simulink model "untitled"  (R2023a)
settings: Solver=VariableStepAuto  StartTime=0.0  StopTime=25  RelTol=1e-3
libraries: simulink x2
settings Model: Creator=4epe3  LastModifiedBy=4epe3

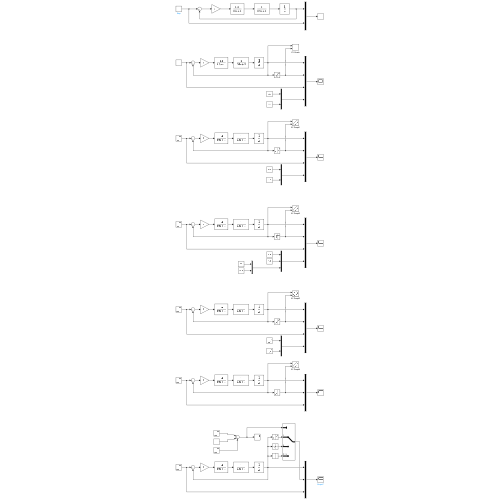
[thumbnail: Simulink's stored preview of the top-level diagram]
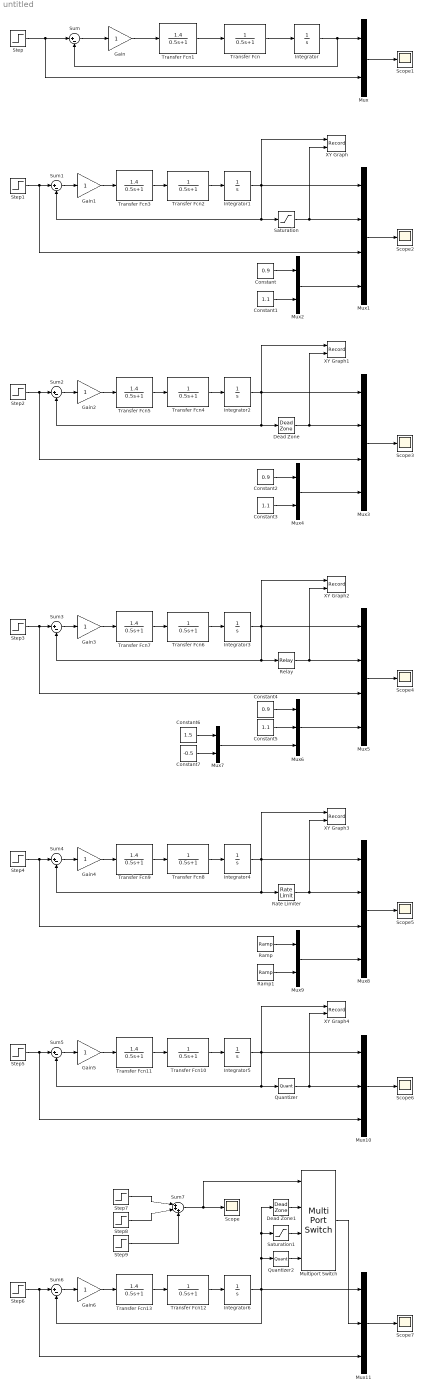
== system untitled ==
  Constant : Constant  Value=0.9
  Constant1 : Constant  Value=1.1
  Constant2 : Constant  Value=0.9
  Constant3 : Constant  Value=1.1
  Constant4 : Constant  Value=0.9
  Constant5 : Constant  Value=1.1
  Constant6 : Constant  Value=1.5
  Constant7 : Constant  Value=-0.5
  Dead Zone : DeadZone  LowerValue=0.9  UpperValue=1.1
  Dead Zone1 : DeadZone  LowerValue=0.9  UpperValue=1.1
  Gain{,1..6} (7 alike) : Gain
  Integrator{,1..6} (7 alike) : Integrator
  Multiport Switch : MultiPortSwitch  SaturateOnIntegerOverflow=off  InputSameDT=off
  Mux{,2,4,7,9} (5 alike) : Mux  Inputs=2
  Mux{1,3,5,8} (4 alike) : Mux
  Mux10 : Mux  Inputs=3
  Mux11 : Mux  Inputs=3
  Mux6 : Mux  Inputs=3
  Quantizer : Quantizer  QuantizationInterval=0.2
  Quantizer2 : Quantizer  QuantizationInterval=0.2
  Ramp : simulink/Sources/Ramp  slope=0.3  start=0  InitialOutput=0
  Ramp1 : simulink/Sources/Ramp  slope=-0.15  start=0  InitialOutput=0
  Rate Limiter : RateLimiter  RisingSlewLimit=0.3  FallingSlewLimit=-0.15  SampleTimeMode=inherited
  Relay : Relay  OnSwitchValue=1.1  OffSwitchValue=0.9  OnOutputValue=1.5  OffOutputValue=-0.5
  Saturation : Saturate  UpperLimit=1.1  LowerLimit=0.9
  Saturation1 : Saturate  UpperLimit=1.1  LowerLimit=0.9
  Scope{,1..7} (8 alike) : Scope
  Step{,1..7} (8 alike) : Step  Time=0  SampleTime=0
  Step8 : Step  Time=10  SampleTime=0
  Step9 : Step  Time=20  SampleTime=0
  Sum{,1..6} (7 alike) : Sum  Inputs=|+-
  Sum7 : Sum  Inputs=|+++
  Transfer Fcn{,2,4,6,8,10,12} (7 alike) : TransferFcn  Denominator=[0.5 1]
  Transfer Fcn{1,3,5,7,9,11,13} (7 alike) : TransferFcn  Numerator=[1.4]  Denominator=[0.5 1]
  XY Graph : Record  FileSettingsInternal="{\"entries\":[{\"content\":{\"excelSettings\":{\"content\":{},\"type\":\"Streamout.ExcelSettings\"}},\"type\":\"Streamout.FileSettingStorage\",\"uuid\":\"\"}],\"packageUris\":[\"http:\\/\\/schema.mathworks.com\\/mf0\\/streamout_blocks\\/R2020a\"],\"version\":\"1.0\"}"  Layout=[1 1]  SignalsInternal="{\"entries\":[{\"content\":{\"signals\":[{\"content\":{\"blockPath\":[],\"dimensions\":[1],\"domain\":\"\",\"lineColor\":\"#a2142f\",\"plots\":[1],\"port\":1,\"sid\":[\"\"],\"signalID\":484,\"signalName\":\"Integrator1\"},\"type\":\"RecordBlkView.Signal\",\"uuid\":\"\"},{\"content\":{\"blockPath\":[],\"dimensions\":[1],\"domain\":\"\",\"lineColor\":\"#139fff\",\"plots\":[1],\"port\":2,\"sid\":[\"\"],\"signalID\":488,\"signalName\":\"Saturation\"},\"type\":\"RecordBlkView.Signal\",\"uuid\":\"\"}]},\"type\":\"RecordBlkView.InputSignals\",\"uuid\":\"\"}],\"packageUris\":[\"http:\\/\\/schema.mathworks.com\\/mf0\\/streamout_blocks\\/R2020a\"],\"version\":\"1.0\"}"  VisualizationBindings="{\"xyplotplugin\":{\"info\":[{\"series\":[{\"bindingParametersList\":[{\"parameter\":\"X-Axis\",\"signalID\":484,\"signalName\":\"Integrator1\"},{\"parameter\":\"Y-Axis\",\"signalID\":488,\"signalName\":\"Saturation\"}],\"seriesID\":15759}],\"subplotID\":1}]}}"  CompatibilityTag=XY
  XY Graph1 : Record  FileSettingsInternal="{\"entries\":[{\"content\":{\"excelSettings\":{\"content\":{},\"type\":\"Streamout.ExcelSettings\"}},\"type\":\"Streamout.FileSettingStorage\",\"uuid\":\"\"}],\"packageUris\":[\"http:\\/\\/schema.mathworks.com\\/mf0\\/streamout_blocks\\/R2020a\"],\"version\":\"1.0\"}"  Layout=[1 1]  SignalsInternal="{\"entries\":[{\"content\":{\"signals\":[{\"content\":{\"blockPath\":[],\"dimensions\":[1],\"domain\":\"\",\"lineColor\":\"#a2142f\",\"plots\":[1],\"port\":1,\"sid\":[\"\"],\"signalID\":492,\"signalName\":\"Integrator2\"},\"type\":\"RecordBlkView.Signal\",\"uuid\":\"\"},{\"content\":{\"blockPath\":[],\"dimensions\":[1],\"domain\":\"\",\"lineColor\":\"#139fff\",\"plots\":[1],\"port\":2,\"sid\":[\"\"],\"signalID\":496,\"signalName\":\"Dead Zone\"},\"type\":\"RecordBlkView.Signal\",\"uuid\":\"\"}]},\"type\":\"RecordBlkView.InputSignals\",\"uuid\":\"\"}],\"packageUris\":[\"http:\\/\\/schema.mathworks.com\\/mf0\\/streamout_blocks\\/R2020a\"],\"version\":\"1.0\"}"  VisualizationBindings="{\"xyplotplugin\":{\"info\":[{\"series\":[{\"bindingParametersList\":[{\"parameter\":\"X-Axis\",\"signalID\":492,\"signalName\":\"Integrator2\"},{\"parameter\":\"Y-Axis\",\"signalID\":496,\"signalName\":\"Dead Zone\"}],\"seriesID\":54169}],\"subplotID\":1}]}}"  CompatibilityTag=XY
  XY Graph2 : Record  FileSettingsInternal="{\"entries\":[{\"content\":{\"excelSettings\":{\"content\":{},\"type\":\"Streamout.ExcelSettings\"}},\"type\":\"Streamout.FileSettingStorage\",\"uuid\":\"\"}],\"packageUris\":[\"http:\\/\\/schema.mathworks.com\\/mf0\\/streamout_blocks\\/R2020a\"],\"version\":\"1.0\"}"  Layout=[1 1]  SignalsInternal="{\"entries\":[{\"content\":{\"signals\":[{\"content\":{\"blockPath\":[],\"dimensions\":[1],\"domain\":\"\",\"lineColor\":\"#a2142f\",\"plots\":[1],\"port\":1,\"sid\":[\"\"],\"signalID\":500,\"signalName\":\"Integrator3\"},\"type\":\"RecordBlkView.Signal\",\"uuid\":\"\"},{\"content\":{\"blockPath\":[],\"dimensions\":[1],\"domain\":\"\",\"lineColor\":\"#139fff\",\"plots\":[1],\"port\":2,\"sid\":[\"\"],\"signalID\":504,\"signalName\":\"Relay\"},\"type\":\"RecordBlkView.Signal\",\"uuid\":\"\"}]},\"type\":\"RecordBlkView.InputSignals\",\"uuid\":\"\"}],\"packageUris\":[\"http:\\/\\/schema.mathworks.com\\/mf0\\/streamout_blocks\\/R2020a\"],\"version\":\"1.0\"}"  VisualizationBindings="{\"xyplotplugin\":{\"info\":[{\"series\":[{\"bindingParametersList\":[{\"parameter\":\"X-Axis\",\"signalID\":500,\"signalName\":\"Integrator3\"},{\"parameter\":\"Y-Axis\",\"signalID\":504,\"signalName\":\"Relay\"}],\"seriesID\":28450}],\"subplotID\":1}]}}"  CompatibilityTag=XY
  XY Graph3 : Record  FileSettingsInternal="{\"entries\":[{\"content\":{\"excelSettings\":{\"content\":{},\"type\":\"Streamout.ExcelSettings\"}},\"type\":\"Streamout.FileSettingStorage\",\"uuid\":\"\"}],\"packageUris\":[\"http:\\/\\/schema.mathworks.com\\/mf0\\/streamout_blocks\\/R2020a\"],\"version\":\"1.0\"}"  Layout=[1 1]  SignalsInternal="{\"entries\":[{\"content\":{\"signals\":[{\"content\":{\"blockPath\":[],\"dimensions\":[1],\"domain\":\"\",\"lineColor\":\"#a2142f\",\"plots\":[1],\"port\":1,\"sid\":[\"\"],\"signalID\":508,\"signalName\":\"Integrator4\"},\"type\":\"RecordBlkView.Signal\",\"uuid\":\"\"},{\"content\":{\"blockPath\":[],\"dimensions\":[1],\"domain\":\"\",\"lineColor\":\"#139fff\",\"plots\":[1],\"port\":2,\"sid\":[\"\"],\"signalID\":512,\"signalName\":\"Rate Limiter\"},\"type\":\"RecordBlkView.Signal\",\"uuid\":\"\"}]},\"type\":\"RecordBlkView.InputSignals\",\"uuid\":\"\"}],\"packageUris\":[\"http:\\/\\/schema.mathworks.com\\/mf0\\/streamout_blocks\\/R2020a\"],\"version\":\"1.0\"}"  VisualizationBindings="{\"xyplotplugin\":{\"info\":[{\"series\":[{\"bindingParametersList\":[{\"parameter\":\"X-Axis\",\"signalID\":508,\"signalName\":\"Integrator4\"},{\"parameter\":\"Y-Axis\",\"signalID\":512,\"signalName\":\"Rate Limiter\"}],\"seriesID\":19812}],\"subplotID\":1}]}}"  CompatibilityTag=XY
  XY Graph4 : Record  FileSettingsInternal="{\"entries\":[{\"content\":{\"excelSettings\":{\"content\":{},\"type\":\"Streamout.ExcelSettings\"}},\"type\":\"Streamout.FileSettingStorage\",\"uuid\":\"\"}],\"packageUris\":[\"http:\\/\\/schema.mathworks.com\\/mf0\\/streamout_blocks\\/R2020a\"],\"version\":\"1.0\"}"  Layout=[1 1]  SignalsInternal="{\"entries\":[{\"content\":{\"signals\":[{\"content\":{\"blockPath\":[],\"dimensions\":[1],\"domain\":\"\",\"lineColor\":\"#a2142f\",\"plots\":[1],\"port\":1,\"sid\":[\"\"],\"signalID\":516,\"signalName\":\"Integrator5\"},\"type\":\"RecordBlkView.Signal\",\"uuid\":\"\"},{\"content\":{\"blockPath\":[],\"dimensions\":[1],\"domain\":\"\",\"lineColor\":\"#139fff\",\"plots\":[1],\"port\":2,\"sid\":[\"\"],\"signalID\":520,\"signalName\":\"Quantizer\"},\"type\":\"RecordBlkView.Signal\",\"uuid\":\"\"}]},\"type\":\"RecordBlkView.InputSignals\",\"uuid\":\"\"}],\"packageUris\":[\"http:\\/\\/schema.mathworks.com\\/mf0\\/streamout_blocks\\/R2020a\"],\"version\":\"1.0\"}"  VisualizationBindings="{\"xyplotplugin\":{\"info\":[{\"series\":[{\"bindingParametersList\":[{\"parameter\":\"X-Axis\",\"signalID\":516,\"signalName\":\"Integrator5\"},{\"parameter\":\"Y-Axis\",\"signalID\":520,\"signalName\":\"Quantizer\"}],\"seriesID\":30653}],\"subplotID\":1}]}}"  CompatibilityTag=XY
  wires:
  Gain/1 -> Transfer Fcn1/1
  Transfer Fcn1/1 -> Transfer Fcn/1
  Sum/1 -> Gain/1
  Transfer Fcn/1 -> Integrator/1
  Integrator/1 -> Mux/1, Sum/2
  Mux/1 -> Scope1/1
  Step/1 -> Sum/1, Mux/2
  Transfer Fcn2/1 -> Integrator1/1
  Sum1/1 -> Gain1/1
  Step1/1 -> Mux1/3, Sum1/1
  Mux1/1 -> Scope2/1
  Gain1/1 -> Transfer Fcn3/1
  Transfer Fcn3/1 -> Transfer Fcn2/1
  Integrator1/1 -> Mux1/1, Saturation/1, Sum1/2, XY Graph/1
  Saturation/1 -> XY Graph/2, Mux1/2
  Constant1/1 -> Mux2/2
  Constant/1 -> Mux2/1
  Mux2/1 -> Mux1/4
  Constant2/1 -> Mux4/1
  Dead Zone/1 -> XY Graph1/2, Mux3/2
  Mux4/1 -> Mux3/4
  Constant3/1 -> Mux4/2
  Integrator2/1 -> Mux3/1, Dead Zone/1, Sum2/2, XY Graph1/1
  Transfer Fcn5/1 -> Transfer Fcn4/1
  Step2/1 -> Mux3/3, Sum2/1
  Sum2/1 -> Gain2/1
  Transfer Fcn4/1 -> Integrator2/1
  Gain2/1 -> Transfer Fcn5/1
  Mux3/1 -> Scope3/1
  Constant4/1 -> Mux6/1
  Relay/1 -> XY Graph2/2, Mux5/2
  Step3/1 -> Mux5/3, Sum3/1
  Transfer Fcn7/1 -> Transfer Fcn6/1
  Integrator3/1 -> Mux5/1, Relay/1, Sum3/2, XY Graph2/1
  Mux6/1 -> Mux5/4
  Sum3/1 -> Gain3/1
  Constant5/1 -> Mux6/2
  Gain3/1 -> Transfer Fcn7/1
  Mux5/1 -> Scope4/1
  Transfer Fcn6/1 -> Integrator3/1
  Mux7/1 -> Mux6/3
  Constant6/1 -> Mux7/1
  Constant7/1 -> Mux7/2
  Ramp/1 -> Mux9/1
  Rate Limiter/1 -> XY Graph3/2, Mux8/2
  Step4/1 -> Mux8/3, Sum4/1
  Transfer Fcn9/1 -> Transfer Fcn8/1
  Integrator4/1 -> Mux8/1, Rate Limiter/1, Sum4/2, XY Graph3/1
  Mux9/1 -> Mux8/4
  Sum4/1 -> Gain4/1
  Ramp1/1 -> Mux9/2
  Gain4/1 -> Transfer Fcn9/1
  Mux8/1 -> Scope5/1
  Transfer Fcn8/1 -> Integrator4/1
  Transfer Fcn11/1 -> Transfer Fcn10/1
  Step5/1 -> Mux10/3, Sum5/1
  Quantizer/1 -> XY Graph4/2, Mux10/2
  Transfer Fcn10/1 -> Integrator5/1
  Mux10/1 -> Scope6/1
  Gain5/1 -> Transfer Fcn11/1
  Sum5/1 -> Gain5/1
  Integrator5/1 -> Mux10/1, Quantizer/1, Sum5/2, XY Graph4/1
  Transfer Fcn12/1 -> Integrator6/1
  Step6/1 -> Mux11/3, Sum6/1
  Sum6/1 -> Gain6/1
  Gain6/1 -> Transfer Fcn13/1
  Integrator6/1 -> Quantizer2/1, Saturation1/1, Dead Zone1/1, Mux11/1, Sum6/2
  Mux11/1 -> Scope7/1
  Transfer Fcn13/1 -> Transfer Fcn12/1
  Step7/1 -> Sum7/1
  Step8/1 -> Sum7/2
  Step9/1 -> Sum7/3
  Sum7/1 -> Multiport Switch/1, Scope/1
  Quantizer2/1 -> Multiport Switch/4
  Multiport Switch/1 -> Mux11/2
  Saturation1/1 -> Multiport Switch/3
  Dead Zone1/1 -> Multiport Switch/2
